simulink model "exp7_120"  (R2024b)
settings: Solver=VariableStepDiscrete  StartTime=0.0  StopTime=5  RelTol=1e-3
libraries: spsIGBTDiodeLib x6, spsThreePhaseVIMeasurementLib x2, spsDCVoltageSourceLib x1, spsGroundLib x1, spsThreePhaseSeriesRLCBranchLib x1, spspowerguiLib x1
settings Model: Creator=rushi  LastModifiedBy=nishthadoshi
settings DataIOCC: ReturnWorkspaceOutputs=off

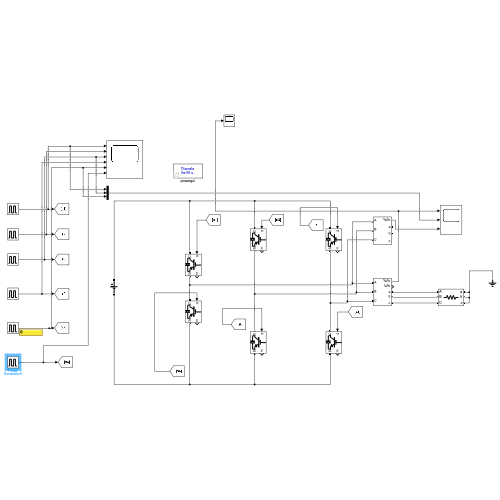
[thumbnail: Simulink's stored preview of the top-level diagram]
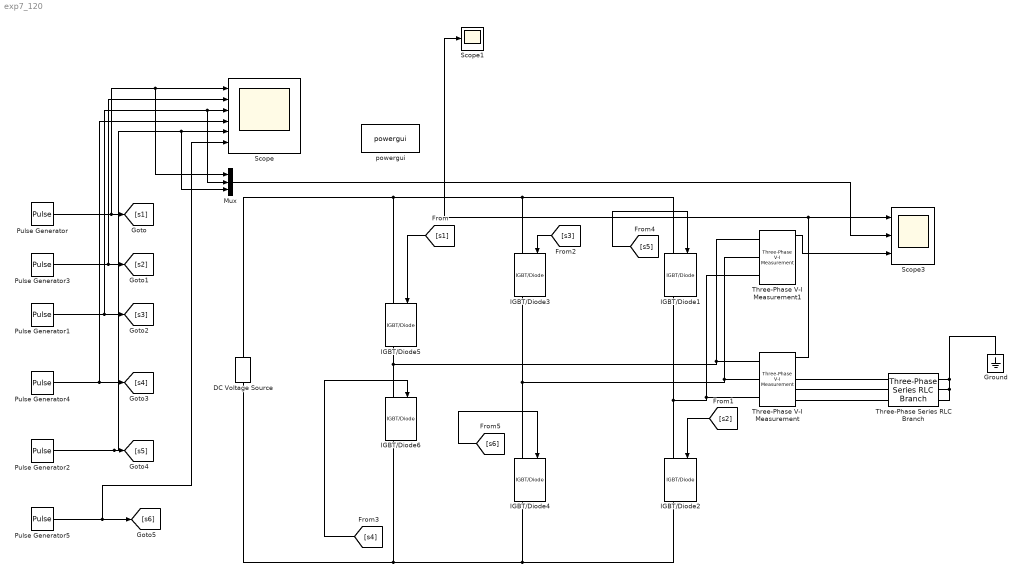
== system exp7_120 ==
  DC Voltage Source : spsDCVoltageSourceLib/DC Voltage Source  Amplitude=100  Measurements=None
  Ground : spsGroundLib/Ground  LConnTagsString=a
  IGBT/Diode{1..6} (6 alike) : spsIGBTDiodeLib/IGBT//Diode  Ron=1e-3  Rs=1e5  Cs=inf  Measurements=on
  Mux : Mux  Inputs=3
  Pulse Generator : DiscretePulseGenerator  PulseType=Time based  Period=0.1  PulseWidth=100/3
  Pulse Generator1 : DiscretePulseGenerator  PulseType=Time based  Period=0.1  PulseWidth=100/3  PhaseDelay=0.1/3
  Pulse Generator2 : DiscretePulseGenerator  PulseType=Time based  Period=0.1  PulseWidth=100/3  PhaseDelay=0.2/3
  Pulse Generator3 : DiscretePulseGenerator  PulseType=Time based  Period=0.1  PulseWidth=100/3  PhaseDelay=0.1/6  VectorParams1D=off
  Pulse Generator4 : DiscretePulseGenerator  PulseType=Time based  Period=0.1  PulseWidth=100/3  PhaseDelay=0.1/2
  Pulse Generator5 : DiscretePulseGenerator  PulseType=Time based  Period=0.1  PulseWidth=100/3  PhaseDelay=0.5/6
  Scope : Scope  NumInputPorts=6
  Scope1 : Scope
  Scope3 : Scope  NumInputPorts=3
  Three-Phase Series RLC Branch : spsThreePhaseSeriesRLCBranchLib/Three-Phase Series RLC Branch  LConnTagsString=A|B|C  RConnTagsString=A|B|C  BranchType=R  Resistance=10  Inductance=1e-3  Capacitance=1e-6  Measurements=None
  Three-Phase V-I Measurement : spsThreePhaseVIMeasurementLib/Three-Phase V-I Measurement  VoltageMeasurement=phase-to-ground  SetLabelV=off  LabelV=Vabc  Vpu=off  VpuLL=off  CurrentMeasurement=yes  SetLabelI=off  LabelI=Iabc  Ipu=off  Pbase=100e6  Vbase=500e3  OutputType=Complex  PhasorSimulation=off  PSBequivalent=0
  Three-Phase V-I Measurement1 : spsThreePhaseVIMeasurementLib/Three-Phase V-I Measurement  VoltageMeasurement=phase-to-phase  SetLabelV=off  LabelV=Vabc  Vpu=off  VpuLL=off  CurrentMeasurement=no  SetLabelI=off  LabelI=Iabc  Ipu=off  Pbase=100e6  Vbase=500e3  OutputType=Complex  PhasorSimulation=off  PSBequivalent=0
  powergui : spspowerguiLib/powergui  Priority=1  SimulationMode=Discrete  SampleTime=5e-6  frequency=60  Iterations=50  frequencyindice=0  Pbase=100e6  ErrMax=1e-4  UnitsV=kV  UnitsW=MW  buscounter=0  FunctionMessages=off  echomessages=off  EnableUseOfTLC=off  CurrentSourceSwitches=off  DisableSnubberDevices=off  DisableRonSwitches=off  DisableVfSwitches=off  DisplayEquations=off  AutomaticDiscreteSolvers=off  SolverType=Tustin/Backward Euler (TBE)  Interpol=off  ExternalGateDelay=off  methode=off  Ts=100  x0status=blocks  SPID=on  SwTol=0  HookPort=off  NonlinearTolerance=1e-4  nMaxIteration=100  ContinueOnMaxIteration=off  RestoreLinks=warning  ResistiveCurrentMeasurement=off  Frange=[0:2:500]  Ylog=off  Xlog=on  ShowGrid=off  save=off  variable=ZData  structure=0  ZoomFFT=off  StartTime=0.0  cycles=1  DisplayStyle=1  fundamental=60  FreqAxis=off  MaxFrequency=1000  frequencyindicesteady=1  RmsSteady=1  display=off
  wires:
  [s1] -> IGBT/Diode5/1
  Pulse Generator/1 -> Mux/1, Scope/1, [s1]
  Pulse Generator1/1 -> Mux/2, Scope/3, [s3]
  Pulse Generator2/1 -> Mux/3, Scope/5, [s5]
  [s3] -> IGBT/Diode3/1
  [s4] -> IGBT/Diode6/1
  [s5] -> IGBT/Diode1/1
  [s6] -> IGBT/Diode4/1
  [s2] -> IGBT/Diode2/1
  Pulse Generator3/1 -> Scope/2, [s2]
  Pulse Generator4/1 -> Scope/4, [s4]
  Pulse Generator5/1 -> Scope/6, [s6]
  Three-Phase V-I Measurement/1 -> Scope3/1, Scope1/1
  Three-Phase V-I Measurement1/1 -> Scope3/3
  Mux/1 -> Scope3/2
  connections:
  DC Voltage Source/RConn1 -- IGBT/Diode5/LConn1 -- IGBT/Diode1/LConn1 -- IGBT/Diode3/LConn1
  IGBT/Diode6/LConn1 -- Three-Phase V-I Measurement1/LConn1 -- Three-Phase V-I Measurement/LConn1 -- IGBT/Diode5/RConn1
  IGBT/Diode4/LConn1 -- Three-Phase V-I Measurement1/LConn2 -- Three-Phase V-I Measurement/LConn2 -- IGBT/Diode3/RConn1
  IGBT/Diode2/LConn1 -- Three-Phase V-I Measurement/LConn3 -- Three-Phase V-I Measurement1/LConn3 -- IGBT/Diode1/RConn1
  IGBT/Diode6/RConn1 -- DC Voltage Source/LConn1 -- IGBT/Diode2/RConn1 -- IGBT/Diode4/RConn1
  Three-Phase Series RLC Branch/LConn1 -- Three-Phase V-I Measurement/RConn1
  Three-Phase Series RLC Branch/LConn2 -- Three-Phase V-I Measurement/RConn2
  Three-Phase Series RLC Branch/LConn3 -- Three-Phase V-I Measurement/RConn3
  Three-Phase Series RLC Branch/RConn1 -- Three-Phase Series RLC Branch/RConn3 -- Three-Phase Series RLC Branch/RConn2 -- Ground/LConn1
